simulink model "Boeing787_OldMission_ElectricalThermalHydraulicFuelECS"  (R2013a)
settings: Solver=ode23tb  SolverMode=SingleTasking  StartTime=0.0  StopTime=346  RelTol=1e-3
InitFcn:
  | load('SampleOutput.mat')
  | 
  | load('SampleFuelBurn.mat')
undefined symbols (not defined in the file or in its folder): ailerons, AirProp, B_737, elevator, FuelBurn, HydProp, landing_gear, rudder, thrust_rev
libraries: PowerFlowLib x118, simulink x20
(part 21 of 26)

== system Boeing787_OldMission_ElectricalThermalHydraulicFuelECS/Electrical/Generation Unit Sync-Sync3/Generator ==
  note: Dynamic model of P.U. Synchronous Generators v1.0
      | Base frequency is 60 Hz
      | Network transients are omitted
      | by Tutku Buyukdegirmenci
  note: Core Dynaimcs
  note: Outputs
  note: Inputs
  note: 0 axis to be implemented
  idq0 : Inport
  w : Inport  Port=2
  ifd' : Inport  Port=3
  Temp : Inport  Port=4
  Demux : Demux  Outputs=3
  Divide : Product  Inputs=*/
  Dynamics : Subsystem
  Electromagnetic Torque Output Power : Subsystem
  Gain1 : Gain  Gain=Xmd/R_fd/VBFD
  Gain2 : Gain  Gain=1/wB
  Gain3 : Gain  Gain=R_fd*VBFD/IBFD
  Gain4 : Gain  Gain=P/2
  Generator Power Loss : Subsystem
  Mux : Mux  Inputs=3
  Product : Product
  Stator Voltage : Subsystem
  Terminator2 : Terminator
  Terminator3 : Terminator
  Terminator4 : Terminator
  V0 : Constant  Value=0
  p.u. transform currents : Gain  Gain=-1/IBDQ
  p.u. transform torque : Gain  Gain=TB
  p.u. transform voltages : Gain  Gain=VBDQ
  vdq0 : Outport
  Te : Outport  Port=2
  vfd' : Outport  Port=3
  Ploss : Outport  Port=4
  wires:
  Gain4/1 -> Gain2/1
  [Efd] -> Dynamics/3(Efd)
  ifd'/1 -> Gain3/1
  idq0/1 -> p.u. transform currents/1
  p.u. transform voltages/1 -> vdq0/1
  Generator Power Loss/3(PLOSS) -> Ploss/1, Terminator4/1
  Generator Power Loss/2(PM) -> Terminator3/1
  Generator Power Loss/1(PE) -> Terminator2/1
  [Te] -> Generator Power Loss/5(Te)
  [nu] -> Generator Power Loss/6(w/ws)
  [Iq] -> Generator Power Loss/4(Iq)
  [Id] -> Generator Power Loss/3(Id)
  [Vq] -> Generator Power Loss/2(Eq)
  [Vd] -> Generator Power Loss/1(Ed)
  p.u. transform torque/1 -> Te/1
  p.u. transform currents/1 -> Demux/1
  [Te] -> p.u. transform torque/1
  Electromagnetic Torque Output Power/1(TE) -> [Te]
  [nu] -> Stator Voltage/7(w/ws)
  V0/1 -> Mux/3
  [Vq] -> Mux/2
  [Vd] -> Mux/1
  Mux/1 -> p.u. transform voltages/1
  [Iq] -> Electromagnetic Torque Output Power/2(Iq), Stator Voltage/2(Iq)
  [Id] -> Electromagnetic Torque Output Power/1(Id), Stator Voltage/1(Id)
  [Iq] -> Dynamics/2(Iq)
  [Id] -> Dynamics/1(Id)
  Gain2/1 -> [nu]
  Demux/2 -> [Iq]
  Demux/1 -> [Id]
  w/1 -> Gain4/1
  Stator Voltage/1(Ed) -> [Vd]
  Stator Voltage/2(Eq) -> [Vq]
  Dynamics/4(Phi_2q) -> Electromagnetic Torque Output Power/6(Phi_2q), Stator Voltage/6(Phi_2q)
  Dynamics/3(Phi_1d) -> Electromagnetic Torque Output Power/5(Phi_1d), Stator Voltage/5(Phi_1d)
  Dynamics/2(Ed1) -> Electromagnetic Torque Output Power/4(Ed1), Stator Voltage/4(Ed1)
  Dynamics/1(Eq1) -> Electromagnetic Torque Output Power/3(Eq1), Stator Voltage/3(Eq1)
  Temp/1 -> [R_temp_delta]
  Gain1/1 -> Divide/1
  Divide/1 -> [Efd]
  Gain3/1 -> Product/1  "vfd'"
  Product/1 -> Gain1/1, vfd'/1
  [R_temp_delta] -> Divide/2, Product/2
  [R_temp_delta] -> Stator Voltage/8(Temp), Dynamics/4(Temp)

== system Boeing787_OldMission_ElectricalThermalHydraulicFuelECS/Electrical/Generation Unit Sync-Sync4/Generator ==
  note: Dynamic model of P.U. Synchronous Generators v1.0
      | Base frequency is 60 Hz
      | Network transients are omitted
      | by Tutku Buyukdegirmenci
  note: Core Dynaimcs
  note: Outputs
  note: Inputs
  note: 0 axis to be implemented
  idq0 : Inport
  w : Inport  Port=2
  ifd' : Inport  Port=3
  Temp : Inport  Port=4
  Demux : Demux  Outputs=3
  Divide : Product  Inputs=*/
  Dynamics : Subsystem
  Electromagnetic Torque Output Power : Subsystem
  Gain1 : Gain  Gain=Xmd/R_fd/VBFD
  Gain2 : Gain  Gain=1/wB
  Gain3 : Gain  Gain=R_fd*VBFD/IBFD
  Gain4 : Gain  Gain=P/2
  Generator Power Loss : Subsystem
  Mux : Mux  Inputs=3
  Product : Product
  Stator Voltage : Subsystem
  Terminator2 : Terminator
  Terminator3 : Terminator
  Terminator4 : Terminator
  V0 : Constant  Value=0
  p.u. transform currents : Gain  Gain=-1/IBDQ
  p.u. transform torque : Gain  Gain=TB
  p.u. transform voltages : Gain  Gain=VBDQ
  vdq0 : Outport
  Te : Outport  Port=2
  vfd' : Outport  Port=3
  Ploss : Outport  Port=4
  wires:
  Gain4/1 -> Gain2/1
  [Efd] -> Dynamics/3(Efd)
  ifd'/1 -> Gain3/1
  idq0/1 -> p.u. transform currents/1
  p.u. transform voltages/1 -> vdq0/1
  Generator Power Loss/3(PLOSS) -> Ploss/1, Terminator4/1
  Generator Power Loss/2(PM) -> Terminator3/1
  Generator Power Loss/1(PE) -> Terminator2/1
  [Te] -> Generator Power Loss/5(Te)
  [nu] -> Generator Power Loss/6(w/ws)
  [Iq] -> Generator Power Loss/4(Iq)
  [Id] -> Generator Power Loss/3(Id)
  [Vq] -> Generator Power Loss/2(Eq)
  [Vd] -> Generator Power Loss/1(Ed)
  p.u. transform torque/1 -> Te/1
  p.u. transform currents/1 -> Demux/1
  [Te] -> p.u. transform torque/1
  Electromagnetic Torque Output Power/1(TE) -> [Te]
  [nu] -> Stator Voltage/7(w/ws)
  V0/1 -> Mux/3
  [Vq] -> Mux/2
  [Vd] -> Mux/1
  Mux/1 -> p.u. transform voltages/1
  [Iq] -> Electromagnetic Torque Output Power/2(Iq), Stator Voltage/2(Iq)
  [Id] -> Electromagnetic Torque Output Power/1(Id), Stator Voltage/1(Id)
  [Iq] -> Dynamics/2(Iq)
  [Id] -> Dynamics/1(Id)
  Gain2/1 -> [nu]
  Demux/2 -> [Iq]
  Demux/1 -> [Id]
  w/1 -> Gain4/1
  Stator Voltage/1(Ed) -> [Vd]
  Stator Voltage/2(Eq) -> [Vq]
  Dynamics/4(Phi_2q) -> Electromagnetic Torque Output Power/6(Phi_2q), Stator Voltage/6(Phi_2q)
  Dynamics/3(Phi_1d) -> Electromagnetic Torque Output Power/5(Phi_1d), Stator Voltage/5(Phi_1d)
  Dynamics/2(Ed1) -> Electromagnetic Torque Output Power/4(Ed1), Stator Voltage/4(Ed1)
  Dynamics/1(Eq1) -> Electromagnetic Torque Output Power/3(Eq1), Stator Voltage/3(Eq1)
  Temp/1 -> [R_temp_delta]
  Gain1/1 -> Divide/1
  Divide/1 -> [Efd]
  Gain3/1 -> Product/1  "vfd'"
  Product/1 -> Gain1/1, vfd'/1
  [R_temp_delta] -> Divide/2, Product/2
  [R_temp_delta] -> Stator Voltage/8(Temp), Dynamics/4(Temp)

== system Boeing787_OldMission_ElectricalThermalHydraulicFuelECS/Electrical/Generation Unit Sync-Sync5/Generator ==
  note: Dynamic model of P.U. Synchronous Generators v1.0
      | Base frequency is 60 Hz
      | Network transients are omitted
      | by Tutku Buyukdegirmenci
  note: Core Dynaimcs
  note: Outputs
  note: Inputs
  note: 0 axis to be implemented
  idq0 : Inport
  w : Inport  Port=2
  ifd' : Inport  Port=3
  Temp : Inport  Port=4
  Demux : Demux  Outputs=3
  Divide : Product  Inputs=*/
  Dynamics : Subsystem
  Electromagnetic Torque Output Power : Subsystem
  Gain1 : Gain  Gain=Xmd/R_fd/VBFD
  Gain2 : Gain  Gain=1/wB
  Gain3 : Gain  Gain=R_fd*VBFD/IBFD
  Gain4 : Gain  Gain=P/2
  Generator Power Loss : Subsystem
  Mux : Mux  Inputs=3
  Product : Product
  Stator Voltage : Subsystem
  Terminator2 : Terminator
  Terminator3 : Terminator
  Terminator4 : Terminator
  V0 : Constant  Value=0
  p.u. transform currents : Gain  Gain=-1/IBDQ
  p.u. transform torque : Gain  Gain=TB
  p.u. transform voltages : Gain  Gain=VBDQ
  vdq0 : Outport
  Te : Outport  Port=2
  vfd' : Outport  Port=3
  Ploss : Outport  Port=4
  wires:
  Gain4/1 -> Gain2/1
  [Efd] -> Dynamics/3(Efd)
  ifd'/1 -> Gain3/1
  idq0/1 -> p.u. transform currents/1
  p.u. transform voltages/1 -> vdq0/1
  Generator Power Loss/3(PLOSS) -> Ploss/1, Terminator4/1
  Generator Power Loss/2(PM) -> Terminator3/1
  Generator Power Loss/1(PE) -> Terminator2/1
  [Te] -> Generator Power Loss/5(Te)
  [nu] -> Generator Power Loss/6(w/ws)
  [Iq] -> Generator Power Loss/4(Iq)
  [Id] -> Generator Power Loss/3(Id)
  [Vq] -> Generator Power Loss/2(Eq)
  [Vd] -> Generator Power Loss/1(Ed)
  p.u. transform torque/1 -> Te/1
  p.u. transform currents/1 -> Demux/1
  [Te] -> p.u. transform torque/1
  Electromagnetic Torque Output Power/1(TE) -> [Te]
  [nu] -> Stator Voltage/7(w/ws)
  V0/1 -> Mux/3
  [Vq] -> Mux/2
  [Vd] -> Mux/1
  Mux/1 -> p.u. transform voltages/1
  [Iq] -> Electromagnetic Torque Output Power/2(Iq), Stator Voltage/2(Iq)
  [Id] -> Electromagnetic Torque Output Power/1(Id), Stator Voltage/1(Id)
  [Iq] -> Dynamics/2(Iq)
  [Id] -> Dynamics/1(Id)
  Gain2/1 -> [nu]
  Demux/2 -> [Iq]
  Demux/1 -> [Id]
  w/1 -> Gain4/1
  Stator Voltage/1(Ed) -> [Vd]
  Stator Voltage/2(Eq) -> [Vq]
  Dynamics/4(Phi_2q) -> Electromagnetic Torque Output Power/6(Phi_2q), Stator Voltage/6(Phi_2q)
  Dynamics/3(Phi_1d) -> Electromagnetic Torque Output Power/5(Phi_1d), Stator Voltage/5(Phi_1d)
  Dynamics/2(Ed1) -> Electromagnetic Torque Output Power/4(Ed1), Stator Voltage/4(Ed1)
  Dynamics/1(Eq1) -> Electromagnetic Torque Output Power/3(Eq1), Stator Voltage/3(Eq1)
  Temp/1 -> [R_temp_delta]
  Gain1/1 -> Divide/1
  Divide/1 -> [Efd]
  Gain3/1 -> Product/1  "vfd'"
  Product/1 -> Gain1/1, vfd'/1
  [R_temp_delta] -> Divide/2, Product/2
  [R_temp_delta] -> Stator Voltage/8(Temp), Dynamics/4(Temp)

== system Boeing787_OldMission_ElectricalThermalHydraulicFuelECS/Electrical/Generation Unit Sync-Sync6/Generator ==
  note: 0 axis to be implemented
  note: Inputs
  note: Outputs
  note: Core Dynaimcs
  note: Dynamic model of P.U. Synchronous Generators v1.0
      | Base frequency is 60 Hz
      | Network transients are omitted
      | by Tutku Buyukdegirmenci
  idq0 : Inport
  w : Inport  Port=2
  ifd' : Inport  Port=3
  Temp : Inport  Port=4
  Demux : Demux  Outputs=3
  Divide : Product  Inputs=*/
  Dynamics : Subsystem
  Electromagnetic Torque Output Power : Subsystem
  Gain1 : Gain  Gain=Xmd/R_fd/VBFD
  Gain2 : Gain  Gain=1/wB
  Gain3 : Gain  Gain=R_fd*VBFD/IBFD
  Gain4 : Gain  Gain=P/2
  Generator Power Loss : Subsystem
  Mux : Mux  Inputs=3
  Product : Product
  Stator Voltage : Subsystem
  Terminator2 : Terminator
  Terminator3 : Terminator
  Terminator4 : Terminator
  V0 : Constant  Value=0
  p.u. transform currents : Gain  Gain=-1/IBDQ
  p.u. transform torque : Gain  Gain=TB
  p.u. transform voltages : Gain  Gain=VBDQ
  vdq0 : Outport
  Te : Outport  Port=2
  vfd' : Outport  Port=3
  Ploss : Outport  Port=4
  wires:
  [R_temp_delta] -> Dynamics/4(Temp), Stator Voltage/8(Temp)
  [R_temp_delta] -> Product/2, Divide/2
  Product/1 -> vfd'/1, Gain1/1
  Gain3/1 -> Product/1  "vfd'"
  Divide/1 -> [Efd]
  Gain1/1 -> Divide/1
  Temp/1 -> [R_temp_delta]
  Dynamics/1(Eq1) -> Stator Voltage/3(Eq1), Electromagnetic Torque Output Power/3(Eq1)
  Dynamics/2(Ed1) -> Stator Voltage/4(Ed1), Electromagnetic Torque Output Power/4(Ed1)
  Dynamics/3(Phi_1d) -> Stator Voltage/5(Phi_1d), Electromagnetic Torque Output Power/5(Phi_1d)
  Dynamics/4(Phi_2q) -> Stator Voltage/6(Phi_2q), Electromagnetic Torque Output Power/6(Phi_2q)
  Stator Voltage/2(Eq) -> [Vq]
  Stator Voltage/1(Ed) -> [Vd]
  w/1 -> Gain4/1
  Demux/1 -> [Id]
  Demux/2 -> [Iq]
  Gain2/1 -> [nu]
  [Id] -> Dynamics/1(Id)
  [Iq] -> Dynamics/2(Iq)
  [Id] -> Stator Voltage/1(Id), Electromagnetic Torque Output Power/1(Id)
  [Iq] -> Stator Voltage/2(Iq), Electromagnetic Torque Output Power/2(Iq)
  Mux/1 -> p.u. transform voltages/1
  [Vd] -> Mux/1
  [Vq] -> Mux/2
  V0/1 -> Mux/3
  [nu] -> Stator Voltage/7(w/ws)
  Electromagnetic Torque Output Power/1(TE) -> [Te]
  [Te] -> p.u. transform torque/1
  p.u. transform currents/1 -> Demux/1
  p.u. transform torque/1 -> Te/1
  [Vd] -> Generator Power Loss/1(Ed)
  [Vq] -> Generator Power Loss/2(Eq)
  [Id] -> Generator Power Loss/3(Id)
  [Iq] -> Generator Power Loss/4(Iq)
  [nu] -> Generator Power Loss/6(w/ws)
  [Te] -> Generator Power Loss/5(Te)
  Generator Power Loss/1(PE) -> Terminator2/1
  Generator Power Loss/2(PM) -> Terminator3/1
  Generator Power Loss/3(PLOSS) -> Terminator4/1, Ploss/1
  p.u. transform voltages/1 -> vdq0/1
  idq0/1 -> p.u. transform currents/1
  ifd'/1 -> Gain3/1
  [Efd] -> Dynamics/3(Efd)
  Gain4/1 -> Gain2/1

== system Boeing787_OldMission_ElectricalThermalHydraulicFuelECS/Fuel/Fuel Tanks//Pumps/FlowGenerator1 ==
  Bias : Bias  Bias=273.15
  Bus Creator1 : BusCreator
  Constant3 : Constant  Value=flowenthalpy
  Constant5 : Constant  Value=flowrate
  Constant6 : Constant  Value=flowtemp
  Constant7 : Constant  Value=flowpres
  FlowOut : Outport  Tag=Flow Out
  wires:
  Bias/1 -> Bus Creator1/2  "temp_K"
  Constant5/1 -> Bus Creator1/1  "mdot_kgps"
  Constant3/1 -> Bus Creator1/4  "H_kJpkg"
  Constant7/1 -> Bus Creator1/3  "pres_kPa"
  Constant6/1 -> Bias/1  "temp_C"
  Bus Creator1/1 -> FlowOut/1  "Outlet"

== system Boeing787_OldMission_ElectricalThermalHydraulicFuelECS/Fuel/Fuel Tanks//Pumps/Fuel Control Left Wing ==
  FuelNeed : Inport
  FuelFromPump : Inport  Port=2
  Bus Creator : BusCreator  Inputs=3
  Bus Creator1 : BusCreator  Inputs=3
  Bus Selector : BusSelector  OutputSignals=mdot_kgps,temp_K,pres_kPa
  Gain : Gain
  Gain1 : Gain
  Saturation : Saturate  UpperLimit=inf  LowerLimit=0
  Sum : Sum  Inputs=|+-
  Switch : Switch  Criteria=u2 > Threshold
  Fuel2Engine : Outport
  Fuel2Tank : Outport  Port=2
  wires:
  Gain1/1 -> Bus Creator1/2  "temp_K"
  Gain/1 -> Bus Creator1/3  "pres_kPa"
  Bus Creator1/1 -> Fuel2Engine/1
  Bus Selector/3 -> Gain/1, Bus Creator/3  "<pres_kPa>"
  Switch/1 -> Bus Creator1/1  "mdot_kgps"
  Saturation/1 -> Bus Creator/1  "mdot_kgps"
  Bus Selector/2 -> Gain1/1, Bus Creator/2  "<temp_K>"
  Bus Creator/1 -> Fuel2Tank/1
  Sum/1 -> Switch/2, Saturation/1
  FuelNeed/1 -> Switch/1, Sum/2
  Bus Selector/1 -> Switch/3, Sum/1  "<mdot_kgps>"
  FuelFromPump/1 -> Bus Selector/1

== system Boeing787_OldMission_ElectricalThermalHydraulicFuelECS/Fuel/Fuel Tanks//Pumps/Fuel Control Right Wing  ==
  FuelNeed : Inport
  FuelFromPump : Inport  Port=2
  Bus Creator : BusCreator  Inputs=3
  Bus Creator1 : BusCreator  Inputs=3
  Bus Selector : BusSelector  OutputSignals=mdot_kgps,temp_K,pres_kPa
  Gain : Gain
  Gain1 : Gain
  Saturation : Saturate  UpperLimit=inf  LowerLimit=0
  Sum : Sum  Inputs=|+-
  Switch : Switch  Criteria=u2 > Threshold
  Fuel2Engine : Outport
  Fuel2Tank : Outport  Port=2
  wires:
  FuelFromPump/1 -> Bus Selector/1
  Bus Selector/1 -> Sum/1, Switch/3  "<mdot_kgps>"
  FuelNeed/1 -> Sum/2, Switch/1
  Sum/1 -> Saturation/1, Switch/2
  Bus Creator/1 -> Fuel2Tank/1
  Bus Selector/2 -> Bus Creator/2, Gain1/1  "<temp_K>"
  Saturation/1 -> Bus Creator/1  "mdot_kgps"
  Switch/1 -> Bus Creator1/1  "mdot_kgps"
  Bus Selector/3 -> Bus Creator/3, Gain/1  "<pres_kPa>"
  Bus Creator1/1 -> Fuel2Engine/1
  Gain/1 -> Bus Creator1/3  "pres_kPa"
  Gain1/1 -> Bus Creator1/2  "temp_K"

== system Boeing787_OldMission_ElectricalThermalHydraulicFuelECS/Fuel/Fuel Tanks//Pumps/Fuel Switch On//Off ==
  Right Wing Tank : Inport
  Center Tank : Inport  Port=2
  Left Wing Tank : Inport  Port=3
  Operating RPM : Constant  Value=6000
  Operating RPM1 : Constant  Value=6000
  Operating RPM2 : Constant  Value=6000
  Right Wing Fuel Pumps On/Off : Switch  Criteria=u2 ~= 0
  Right Wing Fuel Pumps On/Off1 : Switch  Criteria=u2 ~= 0
  Right Wing Fuel Pumps On/Off2 : Switch  Criteria=u2 ~= 0
  shut off : Constant  Value=0
  shut off1 : Constant  Value=0
  shut off2 : Constant  Value=0
  Right Wing RPM : Outport
  Left Wing RPM : Outport  Port=2
  Center RPM : Outport  Port=3
  wires:
  Operating RPM/1 -> Right Wing Fuel Pumps On/Off/1
  shut off/1 -> Right Wing Fuel Pumps On/Off/3
  Right Wing Tank/1 -> Right Wing Fuel Pumps On/Off/2
  Operating RPM1/1 -> Right Wing Fuel Pumps On/Off1/1
  shut off1/1 -> Right Wing Fuel Pumps On/Off1/3
  Center Tank/1 -> Right Wing Fuel Pumps On/Off1/2
  Operating RPM2/1 -> Right Wing Fuel Pumps On/Off2/1
  shut off2/1 -> Right Wing Fuel Pumps On/Off2/3
  Left Wing Tank/1 -> Right Wing Fuel Pumps On/Off2/2
  Right Wing Fuel Pumps On/Off/1 -> Right Wing RPM/1
  Right Wing Fuel Pumps On/Off1/1 -> Center RPM/1
  Right Wing Fuel Pumps On/Off2/1 -> Left Wing RPM/1

== system Boeing787_OldMission_ElectricalThermalHydraulicFuelECS/Fuel/Fuel Tanks//Pumps/Pump Split ==
  Flow In : Inport
  Bus Creator : BusCreator  Inputs=3
  Bus Selector14 : BusSelector  OutputSignals=temp_K,mdot_kgps,pres_kPa
  Gain : Gain  Gain=0.5
  Flow Out : Outport
  wires:
  Bus Selector14/3 -> Bus Creator/3  "<pres_kPa>"
  Gain/1 -> Bus Creator/2  "mdot_kgps"
  Bus Selector14/1 -> Bus Creator/1  "<temp_K>"
  Bus Creator/1 -> Flow Out/1
  Bus Selector14/2 -> Gain/1  "<mdot_kgps>"
  Flow In/1 -> Bus Selector14/1

== system Boeing787_OldMission_ElectricalThermalHydraulicFuelECS/Fuel/Fuel Tanks//Pumps/Pump Split1 ==
  Flow In : Inport
  Bus Creator : BusCreator  Inputs=3
  Bus Selector14 : BusSelector  OutputSignals=temp_K,mdot_kgps,pres_kPa
  Gain : Gain  Gain=0.5
  Flow Out : Outport
  wires:
  Flow In/1 -> Bus Selector14/1
  Bus Selector14/2 -> Gain/1  "<mdot_kgps>"
  Bus Creator/1 -> Flow Out/1
  Bus Selector14/1 -> Bus Creator/1  "<temp_K>"
  Gain/1 -> Bus Creator/2  "mdot_kgps"
  Bus Selector14/3 -> Bus Creator/3  "<pres_kPa>"

== system Boeing787_OldMission_ElectricalThermalHydraulicFuelECS/Fuel/Fuel Tanks//Pumps/Pump Split2 ==
  Flow In : Inport
  Bus Creator : BusCreator  Inputs=3
  Bus Selector14 : BusSelector  OutputSignals=temp_K,mdot_kgps,pres_kPa
  Gain : Gain  Gain=0.5
  Flow Out : Outport
  wires:
  Bus Selector14/3 -> Bus Creator/3  "<pres_kPa>"
  Gain/1 -> Bus Creator/2  "mdot_kgps"
  Bus Selector14/1 -> Bus Creator/1  "<temp_K>"
  Bus Creator/1 -> Flow Out/1
  Bus Selector14/2 -> Gain/1  "<mdot_kgps>"
  Flow In/1 -> Bus Selector14/1

== system Boeing787_OldMission_ElectricalThermalHydraulicFuelECS/Hydraulic/Center Hydraulic System/Bootstrap Reservoir1 ==
  Piston Pressure : Inport
  Bypass Return : Inport  Port=2
  mdot_out : Inport  Port=3
  Return : Inport  Port=4
  Add : Sum  Inputs=+-
  Bleed Valve on/off : Switch  Criteria=u2 ~= 0  ZeroCross=off
  Bleed Valve on/off1 : Switch  Criteria=u2 > Threshold  ZeroCross=off
  Bus Creator : BusCreator  Inputs=2
  Bus Creator1 : BusCreator  Inputs=3
  Bus Creator2 : BusCreator  Inputs=3
  Bus Selector2 : BusSelector  OutputSignals=pres_kPa
  Bus Selector3 : BusSelector  OutputSignals=temp_K,mdot_kgps
  Bus Selector4 : BusSelector  OutputSignals=pres_kPa,mdot_kgps,temp_K
  Divide : Product  Inputs=****/
  Divide1 : Product  Inputs=**/
  Divide2 : Product  Inputs=/*
  Divide3 : Product  Inputs=**
  Divide4 : Product  Inputs=**
  Gain : Gain  Gain=1/1000
  Gain1 : Gain  Gain=pres_loss/100
  Gain{2..7} (6 alike) : Gain
  R_air : Constant  Value=286.9
  Relational Operator : RelationalOperator  OutDataTypeStr=boolean
  Sum : Sum  Inputs=++-
  Sum of Elements : Sum  Inputs=+
  Sum1 : Sum  Inputs=|+-
  Sum2 : Sum  Inputs=-+|
  Sum3 : Sum  Inputs=-+|
  Sum4 : Sum  Inputs=|++
  Temp : Integrator  InitialCondition=T_init  LimitOutput=on  LowerSaturationLimit=eps
  Terminator : Terminator
  Terminator1 : Terminator
  Z(T,P) : Lookup_n-D  BreakpointsForDimension1=AirProp.T2  BreakpointsForDimension2=AirProp.P2  Table=AirProp.Z  RndMeth=Simplest  InputSameDT=on
  air pres : Integrator  InitialCondition=P_init*1000
  mass : Integrator  InitialCondition=mass_init  LimitOutput=on  LowerSaturationLimit=eps
  mass flow off{,1,7..9} (5 alike) : Constant  Value=0
  mass flow off10 : Constant  Value=T_init
  mass flow off2 : Constant  Value=High_Pres_Area
  mass flow off3 : Constant  Value=Low_Pres_Area
  mass flow off4 : Constant  Value=10
  mass flow off5 : Constant  Value=275.79
  mass flow off6 : Constant  Value=-10
  resevor volume : Constant  Value=res_vol
  rho(T) : Lookup_n-D  NumberOfTableDimensions=1  BreakpointsForDimension1=HydProp.T  Table=HydProp.rho_T  RndMeth=Simplest  InputSameDT=on
  Fluid Conditions : Outport
  wires:
  Piston Pressure/1 -> Sum4/1, Divide3/1
  mass flow off1/1 -> Bleed Valve on/off/3
  Divide2/1 -> Sum1/2
  rho(T)/1 -> Divide2/1
  Sum of Elements/1 -> Sum/2
  Return/1 -> Sum of Elements/1
  mass flow off10/1 -> Gain5/1
  Temp/1 -> rho(T)/1, Sum3/1  "temp_K"
  Sum3/1 -> Divide1/1
  Divide1/1 -> Temp/1
  mass/1 -> Divide1/3, Divide2/2
  Bus Creator1/1 -> Fluid Conditions/1
  [valve_cmd] -> Bleed Valve on/off/2
  Relational Operator/1 -> [valve_cmd]
  mass flow off/1 -> Bleed Valve on/off/1
  Bus Selector2/1 -> Relational Operator/1  "<pres_kPa>"
  Bus Selector4/1 -> Relational Operator/2  "<pres_kPa>"
  Bleed Valve on/off/1 -> Terminator1/1, Gain1/1, Sum2/2
  Bus Selector4/2 -> Terminator/1  "<mdot_kgps>"
  Sum2/1 -> Divide/2  "dm/dt"
  Bus Creator/1 -> Bus Selector2/1
  Gain1/1 -> Sum2/1, Bus Creator/1  "mdot_kgps"
  Gain/1 -> Bus Creator/2, Z(T,P)/2  "pres_kPa"
  Sum1/1 -> Divide/5
  resevor volume/1 -> Sum1/1
  air pres/1 -> Gain/1
  Divide/1 -> air pres/1
  Z(T,P)/1 -> Divide/4
  R_air/1 -> Divide/1
  Bus Selector4/3 -> Divide/3, Z(T,P)/1  "<temp_K>"
  Sum/1 -> mass/1  "dm/dt"
  mdot_out/1 -> Gain6/1, Sum/3  "mdot_kgps"
  Bus Selector3/2 -> Sum/1, Divide1/2  "<mdot_kgps>"
  Bypass Return/1 -> Bus Selector3/1
  mass flow off2/1 -> Divide3/2
  mass flow off3/1 -> Divide4/2
  mass flow off5/1 -> Divide4/1
  Divide4/1 -> Add/2
  Divide3/1 -> Add/1
  Add/1 -> Bleed Valve on/off1/2
  mass flow off6/1 -> Bleed Valve on/off1/3
  Bleed Valve on/off1/1 -> Sum4/2
  mass flow off4/1 -> Bleed Valve on/off1/1  "pres_kPa"
  Bus Creator2/1 -> Bus Selector4/1
  mass flow off9/1 -> Gain4/1
  mass flow off8/1 -> Gain3/1
  mass flow off7/1 -> Gain2/1
  Gain2/1 -> Bus Creator2/1  "pres_kPa"
  Gain4/1 -> Bus Creator2/3  "temp_K"
  Gain3/1 -> Bus Creator2/2  "mdot_kgps"
  Gain6/1 -> Bus Creator1/3  "mdot_kgps"
  Gain5/1 -> Bus Creator1/2  "temp_K"
  Sum4/1 -> Gain7/1  "pres_kPa"
  Gain7/1 -> Bus Creator1/1  "pres_kPa"

== system Boeing787_OldMission_ElectricalThermalHydraulicFuelECS/Hydraulic/Center Hydraulic System/Bootstrap Reservoir2 ==
  Piston Pressure : Inport
  Bypass Return : Inport  Port=2
  mdot_out : Inport  Port=3
  Return : Inport  Port=4
  Add : Sum  Inputs=+-
  Bleed Valve on/off : Switch  Criteria=u2 ~= 0  ZeroCross=off
  Bleed Valve on/off1 : Switch  Criteria=u2 > Threshold  ZeroCross=off
  Bus Creator : BusCreator  Inputs=2
  Bus Creator1 : BusCreator  Inputs=3
  Bus Creator2 : BusCreator  Inputs=3
  Bus Selector2 : BusSelector  OutputSignals=pres_kPa
  Bus Selector3 : BusSelector  OutputSignals=temp_K,mdot_kgps
  Bus Selector4 : BusSelector  OutputSignals=pres_kPa,mdot_kgps,temp_K
  Divide : Product  Inputs=****/
  Divide1 : Product  Inputs=**/
  Divide2 : Product  Inputs=/*
  Divide3 : Product  Inputs=**
  Divide4 : Product  Inputs=**
  Gain : Gain  Gain=1/1000
  Gain1 : Gain  Gain=pres_loss/100
  Gain{2..7} (6 alike) : Gain
  R_air : Constant  Value=286.9
  Relational Operator : RelationalOperator  OutDataTypeStr=boolean
  Sum : Sum  Inputs=++-
  Sum of Elements : Sum  Inputs=+
  Sum1 : Sum  Inputs=|+-
  Sum2 : Sum  Inputs=-+|
  Sum3 : Sum  Inputs=-+|
  Sum4 : Sum  Inputs=|++
  Temp : Integrator  InitialCondition=T_init  LimitOutput=on  LowerSaturationLimit=eps
  Terminator : Terminator
  Terminator1 : Terminator
  Z(T,P) : Lookup_n-D  BreakpointsForDimension1=AirProp.T2  BreakpointsForDimension2=AirProp.P2  Table=AirProp.Z  RndMeth=Simplest  InputSameDT=on
  air pres : Integrator  InitialCondition=P_init*1000
  mass : Integrator  InitialCondition=mass_init  LimitOutput=on  LowerSaturationLimit=eps
  mass flow off{,1,7..9} (5 alike) : Constant  Value=0
  mass flow off2 : Constant  Value=High_Pres_Area
  mass flow off3 : Constant  Value=Low_Pres_Area
  mass flow off4 : Constant  Value=10
  mass flow off5 : Constant  Value=275.79
  mass flow off6 : Constant  Value=-10
  resevor volume : Constant  Value=res_vol
  rho(T) : Lookup_n-D  NumberOfTableDimensions=1  BreakpointsForDimension1=HydProp.T  Table=HydProp.rho_T  RndMeth=Simplest  InputSameDT=on
  Fluid Conditions : Outport
  wires:
  Piston Pressure/1 -> Sum4/1, Divide3/1
  mass flow off1/1 -> Bleed Valve on/off/3
  Divide2/1 -> Sum1/2
  rho(T)/1 -> Divide2/1
  Sum of Elements/1 -> Sum/2
  Return/1 -> Sum of Elements/1
  Bus Selector3/1 -> Gain5/1  "<temp_K>"
  Temp/1 -> rho(T)/1, Sum3/1  "temp_K"
  Sum3/1 -> Divide1/1
  Divide1/1 -> Temp/1
  mass/1 -> Divide1/3, Divide2/2
  Bus Creator1/1 -> Fluid Conditions/1
  [valve_cmd] -> Bleed Valve on/off/2
  Relational Operator/1 -> [valve_cmd]
  mass flow off/1 -> Bleed Valve on/off/1
  Bus Selector2/1 -> Relational Operator/1  "<pres_kPa>"
  Bus Selector4/1 -> Relational Operator/2  "<pres_kPa>"
  Bleed Valve on/off/1 -> Terminator1/1, Gain1/1, Sum2/2
  Bus Selector4/2 -> Terminator/1  "<mdot_kgps>"
  Sum2/1 -> Divide/2  "dm/dt"
  Bus Creator/1 -> Bus Selector2/1
  Gain1/1 -> Sum2/1, Bus Creator/1  "mdot_kgps"
  Gain/1 -> Bus Creator/2, Z(T,P)/2  "pres_kPa"
  Sum1/1 -> Divide/5
  resevor volume/1 -> Sum1/1
  air pres/1 -> Gain/1
  Divide/1 -> air pres/1
  Z(T,P)/1 -> Divide/4
  R_air/1 -> Divide/1
  Bus Selector4/3 -> Divide/3, Z(T,P)/1  "<temp_K>"
  Sum/1 -> mass/1  "dm/dt"
  mdot_out/1 -> Gain6/1, Sum/3  "mdot_kgps"
  Bus Selector3/2 -> Sum/1, Divide1/2  "<mdot_kgps>"
  Bypass Return/1 -> Bus Selector3/1
  mass flow off2/1 -> Divide3/2
  mass flow off3/1 -> Divide4/2
  mass flow off5/1 -> Divide4/1
  Divide4/1 -> Add/2
  Divide3/1 -> Add/1
  Add/1 -> Bleed Valve on/off1/2
  mass flow off6/1 -> Bleed Valve on/off1/3
  Bleed Valve on/off1/1 -> Sum4/2
  mass flow off4/1 -> Bleed Valve on/off1/1  "pres_kPa"
  Bus Creator2/1 -> Bus Selector4/1
  mass flow off9/1 -> Gain4/1
  mass flow off8/1 -> Gain3/1
  mass flow off7/1 -> Gain2/1
  Gain2/1 -> Bus Creator2/1  "pres_kPa"
  Gain4/1 -> Bus Creator2/3  "temp_K"
  Gain3/1 -> Bus Creator2/2  "mdot_kgps"
  Gain6/1 -> Bus Creator1/3  "mdot_kgps"
  Gain5/1 -> Bus Creator1/2  "temp_K"
  Sum4/1 -> Gain7/1  "pres_kPa"
  Gain7/1 -> Bus Creator1/1  "pres_kPa"

== system Boeing787_OldMission_ElectricalThermalHydraulicFuelECS/Hydraulic/Center Hydraulic System/DC Speed Servo ==
  T_load (Nm) : Inport
  Speed_ref (RPM) : Inport  Port=2
  Voltage : Inport  Port=3
  DC Machine : Subsystem
  Fcn : Fcn  Expr=u(1)/(u(2)+0.1)
  Gain2 : Gain  Gain=60/(2*pi)
  Mux : Mux  Inputs=2
  PID Controller : simulink/Continuous/PID Controller  Controller=PID  TimeDomain=Continuous-time  SampleTime=1  IntegratorMethod=Forward Euler  FilterMethod=Forward Euler  Form=Parallel  P=1  I=0.1  D=0  N=100  InitialConditionSource=internal  InitialConditionForIntegrator=0  InitialConditionForFilter=0  ExternalReset=none  LimitOutput=off  UpperSaturationLimit=inf  LowerSaturationLimit=-inf  LinearizeAsGain=on  AntiWindupMode=none  Kb=1  TrackingMode=off  Kt=1  PParamMin=[]  PParamMax=[]  IParamMin=[]  IParamMax=[]  DParamMin=[]  DParamMax=[]  NParamMin=[]  NParamMax=[]  KbParamMin=[]  KbParamMax=[]  KtParamMin=[]  KtParamMax=[]  POutMin=[]  POutMax=[]  IOutMin=[]  IOutMax=[]  DOutMin=[]  DOutMax=[]  NOutMin=[]  NOutMax=[]  KbOutMin=[]  KbOutMax=[]  KtOutMin=[]  KtOutMax=[]  IntegratorOutMin=[]  IntegratorOutMax=[]  FilterOutMin=[]  FilterOutMax=[]  SumOutMin=[]  SumOutMax=[]  SumI1OutMin=[]  SumI1OutMax=[]  SumI2OutMin=[]  SumI2OutMax=[]  SumI3OutMin=[]  SumI3OutMax=[]  SumDOutMin=[]  SumDOutMax=[]  SaturationOutMin=[]  SaturationOutMax=[]  IntegratorContinuousStateAttributes=''  IntegratorStateMustResolveToSignalObject=off  IntegratorRTWStateStorageClass=Auto  FilterContinuousStateAttributes=''  FilterStateMustResolveToSignalObject=off  FilterRTWStateStorageClass=Auto
  Sum : Sum  Inputs=-+|
  Terminator{,1..3} (4 alike) : Terminator
  w_m : Outport
  i_load : Outport  Port=2
  T_em : Outport  Port=3
  Ploss : Outport  Port=4
  wires:
  DC Machine/5(Plosses) -> Ploss/1
  Sum/1 -> PID Controller/1
  Gain2/1 -> Sum/1, w_m/1
  Speed_ref (RPM)/1 -> Sum/2
  T_load (Nm)/1 -> DC Machine/3(Tload)
  DC Machine/6(Te) -> T_em/1
  Mux/1 -> Fcn/1
  DC Machine/3(Pe) -> Mux/1
  Fcn/1 -> i_load/1
  DC Machine/7(Speed) -> Gain2/1
  Voltage/1 -> DC Machine/1(Vf), Mux/2
  PID Controller/1 -> DC Machine/2(Va)
  DC Machine/1(If) -> Terminator/1
  DC Machine/2(Ia) -> Terminator1/1
  DC Machine/4(Pm) -> Terminator2/1
  DC Machine/8(theta) -> Terminator3/1

== system Boeing787_OldMission_ElectricalThermalHydraulicFuelECS/Hydraulic/Center Hydraulic System/DC Speed Servo1 ==
  T_load (Nm) : Inport
  Speed_ref (RPM) : Inport  Port=2
  Voltage : Inport  Port=3
  DC Machine : Subsystem
  Fcn : Fcn  Expr=u(1)/(u(2)+0.1)
  Gain2 : Gain  Gain=60/(2*pi)
  Mux : Mux  Inputs=2
  PID Controller : simulink/Continuous/PID Controller  Controller=PID  TimeDomain=Continuous-time  SampleTime=1  IntegratorMethod=Forward Euler  FilterMethod=Forward Euler  Form=Parallel  P=1  I=0.1  D=0  N=100  InitialConditionSource=internal  InitialConditionForIntegrator=0  InitialConditionForFilter=0  ExternalReset=none  LimitOutput=off  UpperSaturationLimit=inf  LowerSaturationLimit=-inf  LinearizeAsGain=on  AntiWindupMode=none  Kb=1  TrackingMode=off  Kt=1  PParamMin=[]  PParamMax=[]  IParamMin=[]  IParamMax=[]  DParamMin=[]  DParamMax=[]  NParamMin=[]  NParamMax=[]  KbParamMin=[]  KbParamMax=[]  KtParamMin=[]  KtParamMax=[]  POutMin=[]  POutMax=[]  IOutMin=[]  IOutMax=[]  DOutMin=[]  DOutMax=[]  NOutMin=[]  NOutMax=[]  KbOutMin=[]  KbOutMax=[]  KtOutMin=[]  KtOutMax=[]  IntegratorOutMin=[]  IntegratorOutMax=[]  FilterOutMin=[]  FilterOutMax=[]  SumOutMin=[]  SumOutMax=[]  SumI1OutMin=[]  SumI1OutMax=[]  SumI2OutMin=[]  SumI2OutMax=[]  SumI3OutMin=[]  SumI3OutMax=[]  SumDOutMin=[]  SumDOutMax=[]  SaturationOutMin=[]  SaturationOutMax=[]  IntegratorContinuousStateAttributes=''  IntegratorStateMustResolveToSignalObject=off  IntegratorRTWStateStorageClass=Auto  FilterContinuousStateAttributes=''  FilterStateMustResolveToSignalObject=off  FilterRTWStateStorageClass=Auto
  Sum : Sum  Inputs=-+|
  Terminator{,1..3} (4 alike) : Terminator
  w_m : Outport
  i_load : Outport  Port=2
  T_em : Outport  Port=3
  Ploss : Outport  Port=4
  wires:
  DC Machine/5(Plosses) -> Ploss/1
  Sum/1 -> PID Controller/1
  Gain2/1 -> Sum/1, w_m/1
  Speed_ref (RPM)/1 -> Sum/2
  T_load (Nm)/1 -> DC Machine/3(Tload)
  DC Machine/6(Te) -> T_em/1
  Mux/1 -> Fcn/1
  DC Machine/3(Pe) -> Mux/1
  Fcn/1 -> i_load/1
  DC Machine/7(Speed) -> Gain2/1
  Voltage/1 -> DC Machine/1(Vf), Mux/2
  PID Controller/1 -> DC Machine/2(Va)
  DC Machine/1(If) -> Terminator3/1
  DC Machine/2(Ia) -> Terminator2/1
  DC Machine/4(Pm) -> Terminator1/1
  DC Machine/8(theta) -> Terminator/1

== system Boeing787_OldMission_ElectricalThermalHydraulicFuelECS/Hydraulic/Center Hydraulic System/Sinks ==
  "Motor PLoss 1 " : Inport
  Motor PLoss 2 : Inport  Port=2
  Motor Current Load 1 : Inport  Port=3
  Motor Current Load 2 : Inport  Port=4
  Out1 : Outport
  wires:
  "Motor PLoss 1 "/1 -> Out1/1

== system Boeing787_OldMission_ElectricalThermalHydraulicFuelECS/Hydraulic/Left Hydraulic System/Bootstrap Reservoir ==
  Piston Pressure : Inport
  Bypass Return : Inport  Port=2
  mdot_out : Inport  Port=3
  Return : Inport  Port=4
  Add : Sum  Inputs=+-
  Bleed Valve on/off : Switch  Criteria=u2 ~= 0  ZeroCross=off
  Bleed Valve on/off1 : Switch  Criteria=u2 > Threshold  ZeroCross=off
  Bus Creator : BusCreator  Inputs=2
  Bus Creator1 : BusCreator  Inputs=3
  Bus Creator2 : BusCreator  Inputs=3
  Bus Selector2 : BusSelector  OutputSignals=pres_kPa
  Bus Selector3 : BusSelector  OutputSignals=temp_K,mdot_kgps
  Bus Selector4 : BusSelector  OutputSignals=pres_kPa,mdot_kgps,temp_K
  Divide : Product  Inputs=****/
  Divide1 : Product  Inputs=**/
  Divide2 : Product  Inputs=/*
  Divide3 : Product  Inputs=**
  Divide4 : Product  Inputs=**
  Gain : Gain  Gain=1/1000
  Gain1 : Gain  Gain=pres_loss/100
  Gain{2..7} (6 alike) : Gain
  R_air : Constant  Value=286.9
  Relational Operator : RelationalOperator  OutDataTypeStr=boolean
  Sum : Sum  Inputs=++-
  Sum of Elements : Sum  Inputs=+
  Sum1 : Sum  Inputs=|+-
  Sum2 : Sum  Inputs=-+|
  Sum3 : Sum  Inputs=-+|
  Sum4 : Sum  Inputs=|++
  Temp : Integrator  InitialCondition=T_init  LimitOutput=on  LowerSaturationLimit=eps
  Terminator : Terminator
  Terminator1 : Terminator
  Z(T,P) : Lookup_n-D  BreakpointsForDimension1=AirProp.T2  BreakpointsForDimension2=AirProp.P2  Table=AirProp.Z  RndMeth=Simplest  InputSameDT=on
  air pres : Integrator  InitialCondition=P_init*1000
  mass : Integrator  InitialCondition=mass_init  LimitOutput=on  LowerSaturationLimit=eps
  mass flow off{,1,7..9} (5 alike) : Constant  Value=0
  mass flow off2 : Constant  Value=High_Pres_Area
  mass flow off3 : Constant  Value=Low_Pres_Area
  mass flow off4 : Constant  Value=10
  mass flow off5 : Constant  Value=275.79
  mass flow off6 : Constant  Value=-10
  resevor volume : Constant  Value=res_vol
  rho(T) : Lookup_n-D  NumberOfTableDimensions=1  BreakpointsForDimension1=HydProp.T  Table=HydProp.rho_T  RndMeth=Simplest  InputSameDT=on
  Fluid Conditions : Outport
  wires:
  Piston Pressure/1 -> Sum4/1, Divide3/1
  mass flow off1/1 -> Bleed Valve on/off/3
  Divide2/1 -> Sum1/2
  rho(T)/1 -> Divide2/1
  Sum of Elements/1 -> Sum/2
  Return/1 -> Sum of Elements/1
  Bus Selector3/1 -> Gain5/1  "<temp_K>"
  Temp/1 -> rho(T)/1, Sum3/1  "temp_K"
  Sum3/1 -> Divide1/1
  Divide1/1 -> Temp/1
  mass/1 -> Divide1/3, Divide2/2
  Bus Creator1/1 -> Fluid Conditions/1
  [valve_cmd] -> Bleed Valve on/off/2
  Relational Operator/1 -> [valve_cmd]
  mass flow off/1 -> Bleed Valve on/off/1
  Bus Selector2/1 -> Relational Operator/1  "<pres_kPa>"
  Bus Selector4/1 -> Relational Operator/2  "<pres_kPa>"
  Bleed Valve on/off/1 -> Terminator1/1, Gain1/1, Sum2/2
  Bus Selector4/2 -> Terminator/1  "<mdot_kgps>"
  Sum2/1 -> Divide/2  "dm/dt"
  Bus Creator/1 -> Bus Selector2/1
  Gain1/1 -> Sum2/1, Bus Creator/1  "mdot_kgps"
  Gain/1 -> Bus Creator/2, Z(T,P)/2  "pres_kPa"
  Sum1/1 -> Divide/5
  resevor volume/1 -> Sum1/1
  air pres/1 -> Gain/1
  Divide/1 -> air pres/1
  Z(T,P)/1 -> Divide/4
  R_air/1 -> Divide/1
  Bus Selector4/3 -> Divide/3, Z(T,P)/1  "<temp_K>"
  Sum/1 -> mass/1  "dm/dt"
  mdot_out/1 -> Gain6/1, Sum/3  "mdot_kgps"
  Bus Selector3/2 -> Sum/1, Divide1/2  "<mdot_kgps>"
  Bypass Return/1 -> Bus Selector3/1
  mass flow off2/1 -> Divide3/2
  mass flow off3/1 -> Divide4/2
  mass flow off5/1 -> Divide4/1
  Divide4/1 -> Add/2
  Divide3/1 -> Add/1
  Add/1 -> Bleed Valve on/off1/2
  mass flow off6/1 -> Bleed Valve on/off1/3
  Bleed Valve on/off1/1 -> Sum4/2
  mass flow off4/1 -> Bleed Valve on/off1/1  "pres_kPa"
  Bus Creator2/1 -> Bus Selector4/1
  mass flow off9/1 -> Gain4/1
  mass flow off8/1 -> Gain3/1
  mass flow off7/1 -> Gain2/1
  Gain2/1 -> Bus Creator2/1  "pres_kPa"
  Gain4/1 -> Bus Creator2/3  "temp_K"
  Gain3/1 -> Bus Creator2/2  "mdot_kgps"
  Gain7/1 -> Bus Creator1/1  "pres_kPa"
  Gain6/1 -> Bus Creator1/3  "mdot_kgps"
  Gain5/1 -> Bus Creator1/2  "temp_K"
  Sum4/1 -> Gain7/1  "pres_kPa"

== system Boeing787_OldMission_ElectricalThermalHydraulicFuelECS/Hydraulic/Left Hydraulic System/Bootstrap Reservoir1 ==
  Piston Pressure : Inport
  Bypass Return : Inport  Port=2
  mdot_out : Inport  Port=3
  Return : Inport  Port=4
  Add : Sum  Inputs=+-
  Bleed Valve on/off : Switch  Criteria=u2 ~= 0  ZeroCross=off
  Bleed Valve on/off1 : Switch  Criteria=u2 > Threshold  ZeroCross=off
  Bus Creator : BusCreator  Inputs=2
  Bus Creator1 : BusCreator  Inputs=3
  Bus Creator2 : BusCreator  Inputs=3
  Bus Selector2 : BusSelector  OutputSignals=pres_kPa
  Bus Selector3 : BusSelector  OutputSignals=temp_K,mdot_kgps
  Bus Selector4 : BusSelector  OutputSignals=pres_kPa,mdot_kgps,temp_K
  Divide : Product  Inputs=****/
  Divide1 : Product  Inputs=**/
  Divide2 : Product  Inputs=/*
  Divide3 : Product  Inputs=**
  Divide4 : Product  Inputs=**
  Gain : Gain  Gain=1/1000
  Gain1 : Gain  Gain=pres_loss/100
  Gain{2..7} (6 alike) : Gain
  R_air : Constant  Value=286.9
  Relational Operator : RelationalOperator  OutDataTypeStr=boolean
  Sum : Sum  Inputs=++-
  Sum of Elements : Sum  Inputs=+
  Sum1 : Sum  Inputs=|+-
  Sum2 : Sum  Inputs=-+|
  Sum3 : Sum  Inputs=-+|
  Sum4 : Sum  Inputs=|++
  Temp : Integrator  InitialCondition=T_init  LimitOutput=on  LowerSaturationLimit=eps
  Terminator : Terminator
  Terminator1 : Terminator
  Z(T,P) : Lookup_n-D  BreakpointsForDimension1=AirProp.T2  BreakpointsForDimension2=AirProp.P2  Table=AirProp.Z  RndMeth=Simplest  InputSameDT=on
  air pres : Integrator  InitialCondition=P_init*1000
  mass : Integrator  InitialCondition=mass_init  LimitOutput=on  LowerSaturationLimit=eps
  mass flow off{,1,7..9} (5 alike) : Constant  Value=0
  mass flow off10 : Constant  Value=T_init
  mass flow off2 : Constant  Value=High_Pres_Area
  mass flow off3 : Constant  Value=Low_Pres_Area
  mass flow off4 : Constant  Value=10
  mass flow off5 : Constant  Value=275.79
  mass flow off6 : Constant  Value=-10
  resevor volume : Constant  Value=res_vol
  rho(T) : Lookup_n-D  NumberOfTableDimensions=1  BreakpointsForDimension1=HydProp.T  Table=HydProp.rho_T  RndMeth=Simplest  InputSameDT=on
  Fluid Conditions : Outport
  wires:
  Piston Pressure/1 -> Sum4/1, Divide3/1
  mass flow off1/1 -> Bleed Valve on/off/3
  Divide2/1 -> Sum1/2
  rho(T)/1 -> Divide2/1
  Sum of Elements/1 -> Sum/2
  Return/1 -> Sum of Elements/1
  mass flow off10/1 -> Gain5/1
  Temp/1 -> rho(T)/1, Sum3/1  "temp_K"
  Sum3/1 -> Divide1/1
  Divide1/1 -> Temp/1
  mass/1 -> Divide1/3, Divide2/2
  Bus Creator1/1 -> Fluid Conditions/1
  [valve_cmd] -> Bleed Valve on/off/2
  Relational Operator/1 -> [valve_cmd]
  mass flow off/1 -> Bleed Valve on/off/1
  Bus Selector2/1 -> Relational Operator/1  "<pres_kPa>"
  Bus Selector4/1 -> Relational Operator/2  "<pres_kPa>"
  Bleed Valve on/off/1 -> Terminator1/1, Gain1/1, Sum2/2
  Bus Selector4/2 -> Terminator/1  "<mdot_kgps>"
  Sum2/1 -> Divide/2  "dm/dt"
  Bus Creator/1 -> Bus Selector2/1
  Gain1/1 -> Sum2/1, Bus Creator/1  "mdot_kgps"
  Gain/1 -> Bus Creator/2, Z(T,P)/2  "pres_kPa"
  Sum1/1 -> Divide/5
  resevor volume/1 -> Sum1/1
  air pres/1 -> Gain/1
  Divide/1 -> air pres/1
  Z(T,P)/1 -> Divide/4
  R_air/1 -> Divide/1
  Bus Selector4/3 -> Divide/3, Z(T,P)/1  "<temp_K>"
  Sum/1 -> mass/1  "dm/dt"
  mdot_out/1 -> Gain6/1, Sum/3  "mdot_kgps"
  Bus Selector3/2 -> Sum/1, Divide1/2  "<mdot_kgps>"
  Bypass Return/1 -> Bus Selector3/1
  mass flow off2/1 -> Divide3/2
  mass flow off3/1 -> Divide4/2
  mass flow off5/1 -> Divide4/1
  Divide4/1 -> Add/2
  Divide3/1 -> Add/1
  Add/1 -> Bleed Valve on/off1/2
  mass flow off6/1 -> Bleed Valve on/off1/3
  Bleed Valve on/off1/1 -> Sum4/2
  mass flow off4/1 -> Bleed Valve on/off1/1  "pres_kPa"
  Bus Creator2/1 -> Bus Selector4/1
  mass flow off9/1 -> Gain4/1
  mass flow off8/1 -> Gain3/1
  mass flow off7/1 -> Gain2/1
  Gain2/1 -> Bus Creator2/1  "pres_kPa"
  Gain4/1 -> Bus Creator2/3  "temp_K"
  Gain3/1 -> Bus Creator2/2  "mdot_kgps"
  Gain7/1 -> Bus Creator1/1  "pres_kPa"
  Gain6/1 -> Bus Creator1/3  "mdot_kgps"
  Gain5/1 -> Bus Creator1/2  "temp_K"
  Sum4/1 -> Gain7/1  "pres_kPa"

== system Boeing787_OldMission_ElectricalThermalHydraulicFuelECS/Hydraulic/Left Hydraulic System/DC Speed Servo ==
  T_load (Nm) : Inport
  Speed_ref (RPM) : Inport  Port=2
  Voltage : Inport  Port=3
  DC Machine : Subsystem
  Fcn : Fcn  Expr=u(1)/(u(2)+0.1)
  Gain2 : Gain  Gain=60/(2*pi)
  Mux : Mux  Inputs=2
  PID Controller : simulink/Continuous/PID Controller  Controller=PID  TimeDomain=Continuous-time  SampleTime=1  IntegratorMethod=Forward Euler  FilterMethod=Forward Euler  Form=Parallel  P=1  I=0.1  D=0  N=100  InitialConditionSource=internal  InitialConditionForIntegrator=0  InitialConditionForFilter=0  ExternalReset=none  LimitOutput=off  UpperSaturationLimit=inf  LowerSaturationLimit=-inf  LinearizeAsGain=on  AntiWindupMode=none  Kb=1  TrackingMode=off  Kt=1  PParamMin=[]  PParamMax=[]  IParamMin=[]  IParamMax=[]  DParamMin=[]  DParamMax=[]  NParamMin=[]  NParamMax=[]  KbParamMin=[]  KbParamMax=[]  KtParamMin=[]  KtParamMax=[]  POutMin=[]  POutMax=[]  IOutMin=[]  IOutMax=[]  DOutMin=[]  DOutMax=[]  NOutMin=[]  NOutMax=[]  KbOutMin=[]  KbOutMax=[]  KtOutMin=[]  KtOutMax=[]  IntegratorOutMin=[]  IntegratorOutMax=[]  FilterOutMin=[]  FilterOutMax=[]  SumOutMin=[]  SumOutMax=[]  SumI1OutMin=[]  SumI1OutMax=[]  SumI2OutMin=[]  SumI2OutMax=[]  SumI3OutMin=[]  SumI3OutMax=[]  SumDOutMin=[]  SumDOutMax=[]  SaturationOutMin=[]  SaturationOutMax=[]  IntegratorContinuousStateAttributes=''  IntegratorStateMustResolveToSignalObject=off  IntegratorRTWStateStorageClass=Auto  FilterContinuousStateAttributes=''  FilterStateMustResolveToSignalObject=off  FilterRTWStateStorageClass=Auto
  Sum : Sum  Inputs=-+|
  Terminator{,1..3} (4 alike) : Terminator
  w_m : Outport
  i_load : Outport  Port=2
  T_em : Outport  Port=3
  Ploss : Outport  Port=4
  wires:
  DC Machine/5(Plosses) -> Ploss/1
  Sum/1 -> PID Controller/1
  Gain2/1 -> Sum/1, w_m/1
  Speed_ref (RPM)/1 -> Sum/2
  T_load (Nm)/1 -> DC Machine/3(Tload)
  DC Machine/6(Te) -> T_em/1
  Mux/1 -> Fcn/1
  DC Machine/3(Pe) -> Mux/1
  Fcn/1 -> i_load/1
  DC Machine/7(Speed) -> Gain2/1
  Voltage/1 -> DC Machine/1(Vf), Mux/2
  PID Controller/1 -> DC Machine/2(Va)
  DC Machine/1(If) -> Terminator/1
  DC Machine/2(Ia) -> Terminator1/1
  DC Machine/4(Pm) -> Terminator2/1
  DC Machine/8(theta) -> Terminator3/1

== system Boeing787_OldMission_ElectricalThermalHydraulicFuelECS/Hydraulic/Left Hydraulic System/Sinks ==
  "Motor PLoss " : Inport
  Motor Current Load : Inport  Port=2
  Out1 : Outport
  wires:
  "Motor PLoss "/1 -> Out1/1

== system Boeing787_OldMission_ElectricalThermalHydraulicFuelECS/Hydraulic/Right Hydraulic System/Bootstrap Reservoir ==
  Piston Pressure : Inport
  Bypass Return : Inport  Port=2
  mdot_out : Inport  Port=3
  Return : Inport  Port=4
  Add : Sum  Inputs=+-
  Bleed Valve on/off : Switch  Criteria=u2 ~= 0  ZeroCross=off
  Bleed Valve on/off1 : Switch  Criteria=u2 > Threshold  ZeroCross=off
  Bus Creator : BusCreator  Inputs=2
  Bus Creator1 : BusCreator  Inputs=3
  Bus Creator2 : BusCreator  Inputs=3
  Bus Selector2 : BusSelector  OutputSignals=pres_kPa
  Bus Selector3 : BusSelector  OutputSignals=temp_K,mdot_kgps
  Bus Selector4 : BusSelector  OutputSignals=pres_kPa,mdot_kgps,temp_K
  Divide : Product  Inputs=****/
  Divide1 : Product  Inputs=**/
  Divide2 : Product  Inputs=/*
  Divide3 : Product  Inputs=**
  Divide4 : Product  Inputs=**
  Gain : Gain  Gain=1/1000
  Gain1 : Gain  Gain=pres_loss/100
  Gain{2..7} (6 alike) : Gain
  R_air : Constant  Value=286.9
  Relational Operator : RelationalOperator  OutDataTypeStr=boolean
  Sum : Sum  Inputs=++-
  Sum of Elements : Sum  Inputs=+
  Sum1 : Sum  Inputs=|+-
  Sum2 : Sum  Inputs=-+|
  Sum3 : Sum  Inputs=-+|
  Sum4 : Sum  Inputs=|++
  Temp : Integrator  InitialCondition=T_init  LimitOutput=on  LowerSaturationLimit=eps
  Terminator : Terminator
  Terminator1 : Terminator
  Z(T,P) : Lookup_n-D  BreakpointsForDimension1=AirProp.T2  BreakpointsForDimension2=AirProp.P2  Table=AirProp.Z  RndMeth=Simplest  InputSameDT=on
  air pres : Integrator  InitialCondition=P_init*1000
  mass : Integrator  InitialCondition=mass_init  LimitOutput=on  LowerSaturationLimit=eps
  mass flow off{,1,7..9} (5 alike) : Constant  Value=0
  mass flow off2 : Constant  Value=High_Pres_Area
  mass flow off3 : Constant  Value=Low_Pres_Area
  mass flow off4 : Constant  Value=10
  mass flow off5 : Constant  Value=275.79
  mass flow off6 : Constant  Value=-10
  resevor volume : Constant  Value=res_vol
  rho(T) : Lookup_n-D  NumberOfTableDimensions=1  BreakpointsForDimension1=HydProp.T  Table=HydProp.rho_T  RndMeth=Simplest  InputSameDT=on
  Fluid Conditions : Outport
  wires:
  Piston Pressure/1 -> Sum4/1, Divide3/1
  mass flow off1/1 -> Bleed Valve on/off/3
  Divide2/1 -> Sum1/2
  rho(T)/1 -> Divide2/1
  Sum of Elements/1 -> Sum/2
  Return/1 -> Sum of Elements/1
  Bus Selector3/1 -> Gain5/1  "<temp_K>"
  Temp/1 -> rho(T)/1, Sum3/1  "temp_K"
  Sum3/1 -> Divide1/1
  Divide1/1 -> Temp/1
  mass/1 -> Divide1/3, Divide2/2
  Bus Creator1/1 -> Fluid Conditions/1
  [valve_cmd] -> Bleed Valve on/off/2
  Relational Operator/1 -> [valve_cmd]
  mass flow off/1 -> Bleed Valve on/off/1
  Bus Selector2/1 -> Relational Operator/1  "<pres_kPa>"
  Bus Selector4/1 -> Relational Operator/2  "<pres_kPa>"
  Bleed Valve on/off/1 -> Terminator1/1, Gain1/1, Sum2/2
  Bus Selector4/2 -> Terminator/1  "<mdot_kgps>"
  Sum2/1 -> Divide/2  "dm/dt"
  Bus Creator/1 -> Bus Selector2/1
  Gain1/1 -> Sum2/1, Bus Creator/1  "mdot_kgps"
  Gain/1 -> Bus Creator/2, Z(T,P)/2  "pres_kPa"
  Sum1/1 -> Divide/5
  resevor volume/1 -> Sum1/1
  air pres/1 -> Gain/1
  Divide/1 -> air pres/1
  Z(T,P)/1 -> Divide/4
  R_air/1 -> Divide/1
  Bus Selector4/3 -> Divide/3, Z(T,P)/1  "<temp_K>"
  Sum/1 -> mass/1  "dm/dt"
  mdot_out/1 -> Gain6/1, Sum/3  "mdot_kgps"
  Bus Selector3/2 -> Sum/1, Divide1/2  "<mdot_kgps>"
  Bypass Return/1 -> Bus Selector3/1
  mass flow off2/1 -> Divide3/2
  mass flow off3/1 -> Divide4/2
  mass flow off5/1 -> Divide4/1
  Divide4/1 -> Add/2
  Divide3/1 -> Add/1
  Add/1 -> Bleed Valve on/off1/2
  mass flow off6/1 -> Bleed Valve on/off1/3
  Bleed Valve on/off1/1 -> Sum4/2
  mass flow off4/1 -> Bleed Valve on/off1/1  "pres_kPa"
  Bus Creator2/1 -> Bus Selector4/1
  mass flow off9/1 -> Gain4/1
  mass flow off8/1 -> Gain3/1
  mass flow off7/1 -> Gain2/1
  Gain2/1 -> Bus Creator2/1  "pres_kPa"
  Gain4/1 -> Bus Creator2/3  "temp_K"
  Gain3/1 -> Bus Creator2/2  "mdot_kgps"
  Gain7/1 -> Bus Creator1/1  "pres_kPa"
  Gain6/1 -> Bus Creator1/3  "mdot_kgps"
  Gain5/1 -> Bus Creator1/2  "temp_K"
  Sum4/1 -> Gain7/1  "pres_kPa"

== system Boeing787_OldMission_ElectricalThermalHydraulicFuelECS/Hydraulic/Right Hydraulic System/Bootstrap Reservoir1 ==
  Piston Pressure : Inport
  Bypass Return : Inport  Port=2
  mdot_out : Inport  Port=3
  Return : Inport  Port=4
  Add : Sum  Inputs=+-
  Bleed Valve on/off : Switch  Criteria=u2 ~= 0  ZeroCross=off
  Bleed Valve on/off1 : Switch  Criteria=u2 > Threshold  ZeroCross=off
  Bus Creator : BusCreator  Inputs=2
  Bus Creator1 : BusCreator  Inputs=3
  Bus Creator2 : BusCreator  Inputs=3
  Bus Selector2 : BusSelector  OutputSignals=pres_kPa
  Bus Selector3 : BusSelector  OutputSignals=temp_K,mdot_kgps
  Bus Selector4 : BusSelector  OutputSignals=pres_kPa,mdot_kgps,temp_K
  Divide : Product  Inputs=****/
  Divide1 : Product  Inputs=**/
  Divide2 : Product  Inputs=/*
  Divide3 : Product  Inputs=**
  Divide4 : Product  Inputs=**
  Gain : Gain  Gain=1/1000
  Gain1 : Gain  Gain=pres_loss/100
  Gain{2..7} (6 alike) : Gain
  R_air : Constant  Value=286.9
  Relational Operator : RelationalOperator  OutDataTypeStr=boolean
  Sum : Sum  Inputs=++-
  Sum of Elements : Sum  Inputs=+
  Sum1 : Sum  Inputs=|+-
  Sum2 : Sum  Inputs=-+|
  Sum3 : Sum  Inputs=-+|
  Sum4 : Sum  Inputs=|++
  Temp : Integrator  InitialCondition=T_init  LimitOutput=on  LowerSaturationLimit=eps
  Terminator : Terminator
  Terminator1 : Terminator
  Z(T,P) : Lookup_n-D  BreakpointsForDimension1=AirProp.T2  BreakpointsForDimension2=AirProp.P2  Table=AirProp.Z  RndMeth=Simplest  InputSameDT=on
  air pres : Integrator  InitialCondition=P_init*1000
  mass : Integrator  InitialCondition=mass_init  LimitOutput=on  LowerSaturationLimit=eps
  mass flow off{,1,7..9} (5 alike) : Constant  Value=0
  mass flow off10 : Constant  Value=T_init
  mass flow off2 : Constant  Value=High_Pres_Area
  mass flow off3 : Constant  Value=Low_Pres_Area
  mass flow off4 : Constant  Value=10
  mass flow off5 : Constant  Value=275.79
  mass flow off6 : Constant  Value=-10
  resevor volume : Constant  Value=res_vol
  rho(T) : Lookup_n-D  NumberOfTableDimensions=1  BreakpointsForDimension1=HydProp.T  Table=HydProp.rho_T  RndMeth=Simplest  InputSameDT=on
  Fluid Conditions : Outport
  wires:
  Piston Pressure/1 -> Sum4/1, Divide3/1
  mass flow off1/1 -> Bleed Valve on/off/3
  Divide2/1 -> Sum1/2
  rho(T)/1 -> Divide2/1
  Sum of Elements/1 -> Sum/2
  Return/1 -> Sum of Elements/1
  mass flow off10/1 -> Gain5/1
  Temp/1 -> rho(T)/1, Sum3/1  "temp_K"
  Sum3/1 -> Divide1/1
  Divide1/1 -> Temp/1
  mass/1 -> Divide1/3, Divide2/2
  Bus Creator1/1 -> Fluid Conditions/1
  [valve_cmd] -> Bleed Valve on/off/2
  Relational Operator/1 -> [valve_cmd]
  mass flow off/1 -> Bleed Valve on/off/1
  Bus Selector2/1 -> Relational Operator/1  "<pres_kPa>"
  Bus Selector4/1 -> Relational Operator/2  "<pres_kPa>"
  Bleed Valve on/off/1 -> Terminator1/1, Gain1/1, Sum2/2
  Bus Selector4/2 -> Terminator/1  "<mdot_kgps>"
  Sum2/1 -> Divide/2  "dm/dt"
  Bus Creator/1 -> Bus Selector2/1
  Gain1/1 -> Sum2/1, Bus Creator/1  "mdot_kgps"
  Gain/1 -> Bus Creator/2, Z(T,P)/2  "pres_kPa"
  Sum1/1 -> Divide/5
  resevor volume/1 -> Sum1/1
  air pres/1 -> Gain/1
  Divide/1 -> air pres/1
  Z(T,P)/1 -> Divide/4
  R_air/1 -> Divide/1
  Bus Selector4/3 -> Divide/3, Z(T,P)/1  "<temp_K>"
  Sum/1 -> mass/1  "dm/dt"
  mdot_out/1 -> Gain6/1, Sum/3  "mdot_kgps"
  Bus Selector3/2 -> Sum/1, Divide1/2  "<mdot_kgps>"
  Bypass Return/1 -> Bus Selector3/1
  mass flow off2/1 -> Divide3/2
  mass flow off3/1 -> Divide4/2
  mass flow off5/1 -> Divide4/1
  Divide4/1 -> Add/2
  Divide3/1 -> Add/1
  Add/1 -> Bleed Valve on/off1/2
  mass flow off6/1 -> Bleed Valve on/off1/3
  Bleed Valve on/off1/1 -> Sum4/2
  mass flow off4/1 -> Bleed Valve on/off1/1  "pres_kPa"
  Bus Creator2/1 -> Bus Selector4/1
  mass flow off9/1 -> Gain4/1
  mass flow off8/1 -> Gain3/1
  mass flow off7/1 -> Gain2/1
  Gain2/1 -> Bus Creator2/1  "pres_kPa"
  Gain4/1 -> Bus Creator2/3  "temp_K"
  Gain3/1 -> Bus Creator2/2  "mdot_kgps"
  Gain6/1 -> Bus Creator1/3  "mdot_kgps"
  Gain5/1 -> Bus Creator1/2  "temp_K"
  Sum4/1 -> Gain7/1  "pres_kPa"
  Gain7/1 -> Bus Creator1/1  "pres_kPa"
